simulink model "ex8_5"  (R2021b)
settings: Solver=VariableStepAuto  StartTime=0.0  StopTime=10.0  FixedStep=1e-4  EnableMultiTasking=on
undefined symbols (not defined in the file or in its folder): a
settings Model: Creator=user  LastModifiedBy=chesterXalan
settings SolverCC: AlgebraicLoopSolver=TrustRegion
settings DataIOCC: LimitDataPoints=on  ReturnWorkspaceOutputs=off
settings OptimizationCC: LifeSpan=inf
settings DebuggingCC: AllowSymbolicDim=off  SFUnexpectedBacktrackingDiag=warning  SFNoUnconditionalDefaultTransitionDiag=warning  SFExecutionAtInitializationDiag=none  SFMachineParentedDataDiag=warning  ArithmeticOperatorsInVariantConditions=warning
settings ModelReferenceCC: PropagateSignalLabelsOutOfModel=off
settings SFSimCC: SimUseLocalCustomCode=off  CustomCodeUndefinedFunction=UseInterfaceOnly
settings RTWCC: RTWUseLocalCustomCode=off
settings CodeAppCC: StateflowObjectComments=on
settings GRTTargetCC: TargetLangStandard=C89/C90 (ANSI)
settings ConfigComp: CovMetricSettings=dw  CovSaveCumulativeToWorkspaceVar=on  CovSaveSingleToWorkspaceVar=on  CovExternalEMLEnable=off

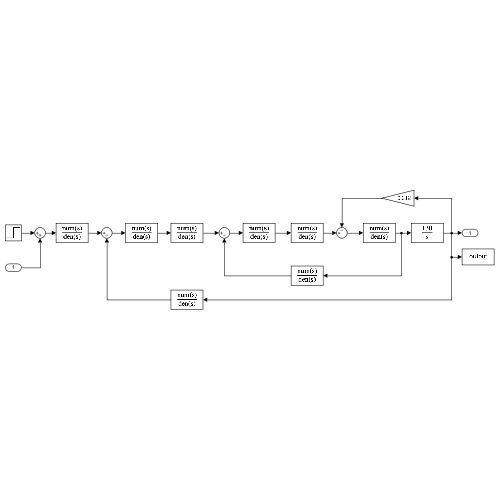
[thumbnail: Simulink's stored preview of the top-level diagram]
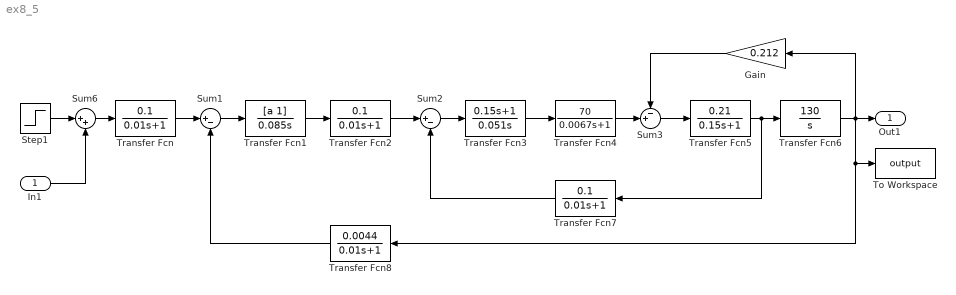
== system ex8_5 ==
  In1 : Inport
  Gain : Gain  Gain=0.212
  Step1 : Step  Time=0.01  SampleTime=1e-3
  Sum1 : Sum  Inputs=|+-
  Sum2 : Sum  Inputs=|+-
  Sum3 : Sum  Inputs=-+|
  Sum6 : Sum  Inputs=|++
  To Workspace : ToWorkspace  VariableName=output  SaveFormat=Timeseries  SampleTime=-1
  Transfer Fcn : TransferFcn  Numerator=[0.1]  Denominator=[0.01 1]
  Transfer Fcn1 : TransferFcn  Numerator=[a 1]  Denominator=[0.085 0]
  Transfer Fcn2 : TransferFcn  Numerator=[0.1]  Denominator=[0.01 1]
  Transfer Fcn3 : TransferFcn  Numerator=[0.15 1]  Denominator=[0.051 0]
  Transfer Fcn4 : TransferFcn  Numerator=[70]  Denominator=[0.0067 1]
  Transfer Fcn5 : TransferFcn  Numerator=[0.21]  Denominator=[0.15 1]
  Transfer Fcn6 : TransferFcn  Numerator=[130]  Denominator=[1 0]
  Transfer Fcn7 : TransferFcn  Numerator=[0.1]  Denominator=[0.01 1]
  Transfer Fcn8 : TransferFcn  Numerator=[0.0044]  Denominator=[0.01 1]
  Out1 : Outport
  wires:
  Step1/1 -> Sum6/1
  Sum1/1 -> Transfer Fcn1/1
  Sum6/1 -> Transfer Fcn/1
  Transfer Fcn/1 -> Sum1/1
  Transfer Fcn1/1 -> Transfer Fcn2/1
  Transfer Fcn2/1 -> Sum2/1
  Transfer Fcn3/1 -> Transfer Fcn4/1
  Transfer Fcn4/1 -> Sum3/2
  Sum2/1 -> Transfer Fcn3/1
  Sum3/1 -> Transfer Fcn5/1
  Transfer Fcn5/1 -> Transfer Fcn7/1, Transfer Fcn6/1
  Gain/1 -> Sum3/1
  In1/1 -> Sum6/2
  Transfer Fcn6/1 -> To Workspace/1, Transfer Fcn8/1, Gain/1, Out1/1
  Transfer Fcn7/1 -> Sum2/2
  Transfer Fcn8/1 -> Sum1/2
